simulink model "Noa_Nofusion"  (R2020b)
settings: Solver=FixedStepDiscrete  StartTime=0.0  StopTime=Inf  FixedStep=0.01  RelTol=1e-3
PostLoadFcn:
  | if any(exist('dsrtsu_mdlpostloadfcn', 'file') ~= 0), dsrtsu_mdlpostloadfcn('Execute', bdroot); end
InitFcn:
  | , if any(exist('rtifpga_mdlclblib', 'file') ~= 0), rtifpga_mdlclblib('Init', bdroot); end,
  | , if any(exist('dsmpb_private', 'file') ~= 0), dsmpb_private('dsmpb_mdlclblib', 'Init', bdroot); end,
undefined symbols (not defined in the file or in its folder): ACC_TimeGap_DecSetSwt, ACC_TimeGap_IncSetSwt, AccelPedalPosn, AccelPedalPosnVldty, AccelPedlPosnDiagc, AccPedalOverride, ACU_ShiftInProgress, ADAS_Posn_CurLane, AESSwtReq, ALC_SwtReq, BrkPedalSts, CC_ACC_CANCEL_OFFSwt, CC_ACC_CRUISE_OFFSwt, CC_ACC_DecSetSpd_SetSwt, CC_ACC_IncSetSpd_ResuSwt, CC_ACCSwtErr, CharSpd_ms, CSA_NODE, CURRENT_GEAR, CurrentGearValid, DiscIntNeverNeededParam, DrvDoorSts, DrvSBR, DrvTrqReqOvld, ECMACCInterface, ECMRespACC, ELKSwtReq, EngLimpHomeSts, EngSpd, EngState, EngState_PHEV, EngTrqMaxActSpd, EngTrqMinAct, EPS_DrvInpTrqVal_HighReslolution, EPS_FailSts, EPS_LKATorqOvrlDlvd, EPS_LKATorqOvrlDlvdVld, EPS_LKATrqOvlDlvdSts, EPS_SteerMod, EPS_TrqSnsrSts, EQ4_APPINFO, EQ4_LA_ELEM, EQ4_LA_HDR, EQ4_LAP_ELEM, EQ4_LAP_HDR, EQ4_LH_ELEM, EQ4_LH_HDR, EQ4_LRE_ELEM, EQ4_LRE_HDR, ESS_PedSwtReq, ESS_VehSwtReq, FFogLmpSts_F_Pbox, FLWheelDriveDirection, FLWheelSpd, FrntWiprSwtSts, FrntWshrSwtSts, FRWheelDriveDirection, FRWheelSpd, HazardLmpSwtSts, HCU_AccelPedalPosn_Diag ... (+151)
libraries: simulink x144, dsmpblib x33, canfdmsglib x10
(part 17 of 20)

== matlab function Noa_Nofusion/TOS2/Subsystem1/ACCOSM/HWA_Task100ms1/VycCalc ==
  data: ObjVyc output single size=15; dxC0 input; aP0 input; bP0 input; aP1 input; bP1 input; ObjValid input boolean size=15; ObjDx input single size=15; ObjVxG input single size=15; ObjVyG input single size=15; ObjYawAngle output
function [ObjVyc,ObjYawAngle] = VycCalc(dxC0,aP0,bP0,aP1,bP1,ObjValid,ObjDx,ObjVxG,ObjVyG)

ObjVyc = single(zeros(15,1));
ObjYawAngle = single(zeros(15,1));

for i=1:15
    if ObjValid(i)
       t_dxv = ObjDx(i);
       t_VxG = ObjVxG(i);
       t_VyG = ObjVyG(i);
       
       if abs(t_VxG)<0.1
          if t_VyG>0.5
              ObjYawAngle(i) = single(1.57);
          end
          if t_VyG<-0.5
              ObjYawAngle(i) = single(-1.57);
          end
       else
           if t_VxG>0
               ObjYawAngle(i) = atan(t_VyG/t_VxG);
           else
               if t_VyG>0
                  ObjYawAngle(i) = single(3.1416) + atan(t_VyG/t_VxG);
               else
                  ObjYawAngle(i) = -single(3.1416) + atan(t_VyG/t_VxG);
               end
           end
       end
       
       t_bParabolaYNLane = single(1);
       if t_dxv<dxC0
          temp1 =  2*aP0*t_dxv + bP0;
          t_bParabolaXNLane = -temp1;
       else
          temp1 =  2*aP1*t_dxv + bP1;
          t_bParabolaXNLane = -temp1;
       end
       t_bParabolaMag = mag(t_bParabolaXNLane,t_bParabolaYNLane);
       t_bParabolaXNLane = t_bParabolaXNLane/t_bParabolaMag;
       t_bParabolaYNLane = t_bParabolaYNLane/t_bParabolaMag;
       temp1 = t_VxG*t_bParabolaXNLane;
       temp2 = t_VyG*t_bParabolaYNLane;
       
       ObjVyc(i) = temp1 + temp2;
    else
       ObjVyc(i) = single(0);
    end
end
end

function out = mag(x,y)
M = max(abs(x),abs(y));
N = min(abs(x),abs(y));
out = M + 0.322*N;
end

== matlab function Noa_Nofusion/TOS2/Subsystem1/ACCOSM/HWA_Task100ms1/dyLaneWidthSteerAdapt ==
  data: kap input; dyLaneAdaptLeft output; dyAdapt input; dyLaneAdaptRight output
function [dyLaneAdaptLeft,dyLaneAdaptRight] = fcn(kap,dyAdapt)

dyLaneAdaptLeft = single(0);
dyLaneAdaptRight = single(0);
if kap>0
    dyLaneAdaptRight = dyAdapt;
end
if kap<0
    dyLaneAdaptLeft = dyAdapt;
end

== matlab function Noa_Nofusion/TOS2/Subsystem1/ACCOSM/HWA_Task100ms1/wCutInVy ==
  data: DycASI output single; ObjValid input boolean size=15; ObjDycCutIn input single size=15; ObjWidth input single size=15; ObjVyc input single size=15; ObjDx input single size=15; ObjDy input single size=15; ObjCnt input uint8 size=15; ObjDycFilt input single size=15; ObjwCutInVyK1 input single size=15; ObjtPrediction4CutIn output single size=15; ObjDycCutInPredict output single size=15; ObjCutIn_b output boolean size=15; ObjwCutInVy output single size=15
function [DycASI,ObjtPrediction4CutIn,ObjDycCutInPredict,ObjCutIn_b,ObjwCutInVy] = ...
    CalcWCutInVy(ObjValid,ObjDycCutIn,ObjWidth,ObjVyc,ObjDx,ObjDy,ObjCnt,...
    ObjDycFilt,ObjwCutInVyK1)
 
ObjwCutInVy = single(zeros(15,1));
ObjtPrediction4CutIn = single(zeros(15,1));
ObjDycCutInPredict = single(zeros(15,1));
DycASI = single(zeros(15,1));
ObjCutIn_b = false(15,1);
 
for i=1:15
    if ObjValid(i)
        dWidth = ObjWidth(i);
        dycASI = ObjDycCutIn(i);
        vyc = ObjVyc(i);
        dx = ObjDx(i);
        dy = ObjDy(i);
        dycFilt = ObjDycFilt(i);
        wCutInVyK1 = ObjwCutInVyK1(i);
  
        temp1 = dycFilt - dycASI;
        if ((dycASI>0)&&(temp1>0.2))||((dycASI<0)&&(temp1<-0.2))
            tauVy = single(1.6);
        else
            tauVy = single(0);
        end
        tauVy = interpolate(single(40),tauVy,single(70),single(0),dx);
        ObjtPrediction4CutIn(i) = tauVy;
        temp1 = vyc*tauVy;
        temp2 = dycASI + temp1;
        
        if (dycASI>0)&&(temp2<0)
            temp2 = single(0);
        else
            if (dycASI<0)&&(temp2>0)
                temp2 = single(0);
            else
                if dycASI==0
                    temp2 = single(0);
                end
            end
        end
        ObjDycCutInPredict(i) = temp2;
        if dycASI>0
            temp1 = temp2 - 0.5*dWidth;
            t_dycASI = max(temp1,single(0));
        else
            temp1 = temp2 + 0.5*dWidth;
            t_dycASI = min(temp1,single(0));
        end
        temp1 = abs(t_dycASI);
        t_wCutInVy = interpolate(single(0),single(1),single(0.7),single(0),temp1);
        if tauVy==0
            t_wCutInVy = single(0);
        end
        
        if dx>0
            fak = abs(dy)/dx; 
        else
            fak = single(0);
        end
        if (ObjCnt(i)<2)||(abs(dy)>=2.4)||(fak>0.25)
           t_wCutInVy = single(0);
        end
       
        temp1 = t_wCutInVy - wCutInVyK1;
        temp1_ub = abs(temp1);
        temp2 = 0.2*temp1_ub;
        if temp1>0
            t_wCutInVy = wCutInVyK1 + temp2;
        else
            t_wCutInVy = wCutInVyK1 - temp2;
        end
        ObjwCutInVy(i) = t_wCutInVy;
        DycASI(i) = t_dycASI;
        if t_wCutInVy>0.7
            ObjCutIn_b(i) = true;
        end
    end
end
end
 
% function out = interpolate(x1,z1,x2,z2,Raw)
% if Raw<=x1
%     out = z1;
% else
%     if Raw>=x2
%         out = z2;
%     else
%         out = z1 + (Raw-x1)*(z2-z1)/(x2-x1);
%     end
% end
% end

== matlab function Noa_Nofusion/TOS2/Subsystem1/ACCOSM/HWA_Task100ms1/wCutOutVy ==
  data: vRef input single size=1; kap input single size=1; tDirIndLeft input single size=1; tDirIndRight input single size=1; ObjValid input boolean size=15; ObjDycCutIn input single size=15; ObjWidth input single size=15; ObjtPrediction4CutOut output single size=15; ObjDycCutOutPredict output single size=15; ObjwCutOutTurnOff output single size=15; ObjVyc input single size=15; ObjDx input single size=15; ObjDy input single size=15; ObjVx input single size=15; ObjVy input single size=15; ObjDyc input single size=15; ObjDrive_b input boolean size=15; ObjCnt input uint8 size=15; ObjDycFilt input single size=15; ObjwCutoutVyK1 input single size=15; ObjwCutoutVy output single size=15
function [ObjtPrediction4CutOut,ObjDycCutOutPredict,ObjwCutOutTurnOff,ObjwCutoutVy] = ...
    CalcWCutOutVy(vRef,kap,tDirIndLeft,tDirIndRight,ObjValid,ObjDycCutIn,ObjWidth,...
    ObjVyc,ObjDx,ObjDy,ObjVx,ObjVy,ObjDyc,ObjDrive_b,ObjCnt,...
    ObjDycFilt,ObjwCutoutVyK1)
 
ObjwCutoutVy = single(zeros(15,1));
ObjtPrediction4CutOut = single(zeros(15,1));
ObjDycCutOutPredict = single(zeros(15,1));
ObjwCutOutTurnOff = single(zeros(15,1));
 
for i=1:15
    if ObjValid(i)
        dWidth = ObjWidth(i);
        dycASI = ObjDycCutIn(i);
        vyc = ObjVyc(i);
        dx = ObjDx(i);
        dy = ObjDy(i);
        vx = ObjVx(i);
        vy = ObjVy(i);
        dyc = ObjDyc(i);
        dycFilt = ObjDycFilt(i);
        wCutoutVyK1 = ObjwCutoutVyK1(i);
        Move_b = ObjDrive_b(i);
        Cnt = ObjCnt(i);
        t_vxTO = vRef + vx;
        t_vxvThreshold = 0.5 - vRef;
        
        temp1 = dycASI - dycFilt;
        if ((dycASI>0)&&(temp1>0.2))||((dycASI<0)&&(temp1<-0.2))
            tauVy = single(1);
        else
            tauVy = single(0);
        end
        tauVy = interpolate(single(40),tauVy,single(70),single(0),dx);
        ObjtPrediction4CutOut(i) = tauVy;
        temp1 = vyc*tauVy;
        temp2 = dycASI + temp1;
        
        if (dycASI>0)&&(temp2<0)
            temp2 = single(0);
        else
            if (dycASI<0)&&(temp2>0)
                temp2 = single(0);
            else
                if dycASI==0
                    temp2 = single(0);
                end
            end
        end
        ObjDycCutOutPredict(i) = temp2;
        if dycASI>0
            temp1 = temp2 + 0.5*dWidth;
            t_dycASI = max(temp1,single(0));
        else
            temp1 = temp2 - 0.5*dWidth;
            t_dycASI = min(temp1,single(0));
        end
        temp1 = abs(t_dycASI);
        t_wCutoutVy = interpolate(single(0),single(0),single(0.7),single(1),temp1);
        if tauVy==0
            t_wCutoutVy = single(0);
        end
        
        temp1 = t_wCutoutVy - wCutoutVyK1;
        temp1_ub = abs(temp1);
        temp2 = 0.2*temp1_ub;
        if temp1>0
            t_wCutoutVy = wCutoutVyK1 + temp2;
        else
            t_wCutoutVy = wCutoutVyK1 - temp2;
        end
        ObjwCutoutVy(i) = t_wCutoutVy;
        if (dx<30)&&(Move_b==true)&&(vRef>0.5)&&(t_vxTO<6)&&(vx>t_vxvThreshold)&&(abs(dyc)>0.5)&&...
        (abs(dy)>0.5)&&(abs(dy)<4)&&(abs(vy)>0.5)&&...
        (((dyc<0)&&(vyc<0)&&(tDirIndRight==0))||((dyc>0)&&(vyc>0)&&(tDirIndLeft==0)))&&...
        (kap>-0.005)&&(kap<0.005)&&...
        (Cnt==7) 
             ObjwCutOutTurnOff(i) = t_wCutoutVy;
        end
    end
end
end

== matlab function Noa_Nofusion/TOS2/Subsystem1/ACCOSM/ObjMatrixTransit/Subsystem/MATLAB Function1 ==
  data: P output uint8; Count input uint8 size=1; ID input uint8 size=20; BrakeLight_b input uint8 size=20; Class input uint8 size=20; LatDis input single size=20; LatVel input single size=20; LongAccel input single size=20; LongDis input single size=20; LongVel input single size=20; Width input single size=20; Age input uint16 size=20; MotionSts input uint8 size=20; ObjValid output boolean size=20; ObjBrakeLightIndic output uint8 size=20; ObjClassification output uint8 size=20; ObjLatPos output single size=20; ObjLatVel output single size=20; ObjLongAccel output single size=20; ObjLongVel output single size=20; ObjWidth output single size=20; ObjCnt output uint8 size=20; ObjMoveSts output uint8 size=20; ObjLongPos output single size=20; ObjIDK1 input uint8 size=20; ObjID output uint8 size=20
function [P,ObjValid,ObjBrakeLightIndic,ObjClassification,...
    ObjLatPos,ObjLatVel,ObjLongAccel,ObjLongVel,...
    ObjWidth,ObjCnt,ObjMoveSts,ObjLongPos,ObjID] =...
    DataT(Count,ID,BrakeLight_b,Class,LatDis,LatVel,LongAccel,LongDis,LongVel,Width,Age,MotionSts,ObjIDK1)

ObjValid = false(20,1);
ObjID = uint8(zeros(20,1));
ObjBrakeLightIndic = uint8(zeros(20,1));
ObjClassification = uint8(zeros(20,1));
ObjLatPos = single(zeros(20,1));
ObjLatVel = single(zeros(20,1));
ObjLongAccel = single(zeros(20,1));
ObjLongPos = single(zeros(20,1));
ObjLongVel = single(zeros(20,1));
ObjWidth = single(zeros(20,1));
ObjCnt = uint8(zeros(20,1));
ObjMoveSts = uint8(zeros(20,1));

T = uint8(zeros(20,1));
P = uint8(zeros(20,1));
Index01 = uint8(zeros(20,1));
Index02 = uint8(zeros(20,1));
M = uint8(0);
N = uint8(0);
w = uint8(0);

for i=uint8(1):Count
    for j=uint8(1):uint8(20)
        if ID(i)==ObjIDK1(j)
            T(j) = i;
            P(i) = j;
        end
    end
end

for j=uint8(1):uint8(20)
    if T(j)==uint8(0)
        if ObjIDK1(j)==uint8(0)
            N = N + uint8(1);
            Index01(N) = j;
        else
            M = M + uint8(1);
            Index02(M) = j;
        end
        ObjValid(j) = false;
    else
        ObjValid(j) = true;
    end
end

for i=uint8(1):Count
    if P(i)==uint8(0)
        w = w + uint8(1);
        if w<=N
            P(i) = Index01(w);
        else
            P(i) = Index02(w - N);
        end
        ObjValid(Index01(w)) = true;
    end
    ObjID(P(i)) = ID(i);
    if BrakeLight_b(i)==uint8(1)
        ObjBrakeLightIndic(P(i)) = uint8(2);
    end
    if Class(i)==uint8(1)||Class(i)==uint8(2)||...
            Class(i)==uint8(3)||Class(i)==uint8(6)
        ObjClassification(P(i)) = uint8(1);
    end
    ObjLatPos(P(i)) = -LatDis(i) - single(0.1);
    ObjLatVel(P(i)) = -LatVel(i);
    ObjLongAccel(P(i)) = LongAccel(i);
    ObjLongPos(P(i)) = LongDis(i);
    ObjLongVel(P(i)) = LongVel(i);
    ObjWidth(P(i)) = Width(i);
    if Age(i)<=255
        ObjCnt(P(i)) = uint8(Age(i)/2) - uint8(1);
    else
        ObjCnt(P(i)) = uint8(127);
    end
    if MotionSts(i)==uint8(1)||MotionSts(i)==uint8(3)
        ObjMoveSts(P(i)) = uint8(1);
    elseif MotionSts(i)==uint8(2)||MotionSts(i)==uint8(5)
        if LongVel(i)>-2.5
            ObjMoveSts(P(i)) = uint8(2);
        else
            ObjMoveSts(P(i)) = uint8(4);
        end
    elseif MotionSts(i)==uint8(4)
        ObjMoveSts(P(i)) = uint8(3);
    end
end
end

== matlab function Noa_Nofusion/Chassis1/CheckSum8Bclc4 ==
  data: Data input; MsgByte output; DataID input
function MsgByte  = CheckSum8B(Data,DataID)
CRC_8_H1D_Tbl =[ 0x00, 0x1d, 0x3a, 0x27, 0x74, 0x69, 0x4e, 0x53, 0xe8, 0xf5, 0xd2, 0xcf, 0x9c, 0x81, 0xa6, 0xbb,...
    0xcd, 0xd0, 0xf7, 0xea, 0xb9, 0xa4, 0x83, 0x9e, 0x25, 0x38, 0x1f, 0x02, 0x51, 0x4c, 0x6b, 0x76, 0x87, 0x9a, 0xbd, 0xa0, 0xf3, 0xee, 0xc9, 0xd4,...
    0x6f, 0x72, 0x55, 0x48, 0x1b, 0x06, 0x21, 0x3c, 0x4a, 0x57, 0x70, 0x6d, 0x3e, 0x23, 0x04, 0x19, 0xa2, 0xbf, 0x98, 0x85, 0xd6, 0xcb, 0xec, 0xf1,...
    0x13, 0x0e, 0x29, 0x34, 0x67, 0x7a, 0x5d, 0x40, 0xfb, 0xe6, 0xc1, 0xdc, 0x8f, 0x92, 0xb5, 0xa8, 0xde, 0xc3, 0xe4, 0xf9, 0xaa, 0xb7, 0x90, 0x8d,...
    0x36, 0x2b, 0x0c, 0x11, 0x42, 0x5f, 0x78, 0x65, 0x94, 0x89, 0xae, 0xb3, 0xe0, 0xfd, 0xda, 0xc7, 0x7c, 0x61, 0x46, 0x5b, 0x08, 0x15, 0x32, 0x2f,...
    0x59, 0x44, 0x63, 0x7e, 0x2d, 0x30, 0x17, 0x0a, 0xb1, 0xac, 0x8b, 0x96, 0xc5, 0xd8, 0xff, 0xe2, 0x26, 0x3b, 0x1c, 0x01, 0x52, 0x4f, 0x68, 0x75,...
    0xce, 0xd3, 0xf4, 0xe9, 0xba, 0xa7, 0x80, 0x9d, 0xeb, 0xf6, 0xd1, 0xcc, 0x9f, 0x82, 0xa5, 0xb8, 0x03, 0x1e, 0x39, 0x24, 0x77, 0x6a, 0x4d, 0x50,...
    0xa1, 0xbc, 0x9b, 0x86, 0xd5, 0xc8, 0xef, 0xf2, 0x49, 0x54, 0x73, 0x6e, 0x3d, 0x20, 0x07, 0x1a, 0x6c, 0x71, 0x56, 0x4b, 0x18, 0x05, 0x22, 0x3f,...
    0x84, 0x99, 0xbe, 0xa3, 0xf0, 0xed, 0xca, 0xd7, 0x35, 0x28, 0x0f, 0x12, 0x41, 0x5c, 0x7b, 0x66, 0xdd, 0xc0, 0xe7, 0xfa, 0xa9, 0xb4, 0x93, 0x8e,...
    0xf8, 0xe5, 0xc2, 0xdf, 0x8c, 0x91, 0xb6, 0xab, 0x10, 0x0d, 0x2a, 0x37, 0x64, 0x79, 0x5e, 0x43, 0xb2, 0xaf, 0x88, 0x95, 0xc6, 0xdb, 0xfc, 0xe1,...
    0x5a, 0x47, 0x60, 0x7d, 0x2e, 0x33, 0x14, 0x09, 0x7f, 0x62, 0x45, 0x58, 0x0b, 0x16, 0x31, 0x2c, 0x97, 0x8a, 0xad, 0xb0, 0xe3, 0xfe, 0xd9, 0xc4];

Segment=uint8(zeros(1,8));

for SegIndex =1:8
    CRC_temp=uint8(0);
    for index = 1:8
        Segment(index)=Data((SegIndex-1)*8+index);
    end
    for index = 1:2
        CRC_temp = bitxor(DataID(SegIndex,index),CRC_temp);
        index1=uint16(CRC_temp)+1;
        CRC_temp = CRC_8_H1D_Tbl(index1);
    end
    for index = 2:8
        CRC_temp = bitxor(Segment(index),CRC_temp);
        index2=uint16(CRC_temp)+1;
        CRC_temp = CRC_8_H1D_Tbl(index2);
    end
    Data(8*SegIndex-7)=CRC_temp;
end
MsgByte=Data;
end

== stateflow chart Noa_Nofusion/TOS2/Subsystem1/ACCOSM/ObjMatrixTransit/Subsystem/Obj ==
  (default) -> (junction 5)
  (junction 5) -> (junction 36) : {i=1;}
  (junction 36) -> (junction 38) [order 1] : [i<21]
  (junction 40) -> (junction 36) : {i=i+1;}
  (junction 36) -> (junction 42) [order 2]
  (junction 38) -> (junction 40) : {id(i) = IFV410_Obj(i).OBJ_ID;
      | confidence(i) = IFV410_Obj(i).OBJ_Existence_Probability;
      | classification(i) = IFV410_Obj(i).OBJ_Object_Class;
      | width(i) = IFV410_Obj(i).OBJ_Width;
      | LongDis(i) = IFV410_Obj(i).OBJ_Long_Distance;
      | LatDis(i) = IFV410_Obj(i).OBJ_Lat_Distance;
      | AbsLongAcc(i) = IFV410_Obj(i).OBJ_Abs_Long_Acc;
      | AbsLongVel(i) = IFV410_Obj(i).OBJ_Abs_Long_Velocity;
      | AbsLatVel(i) = IFV410_Obj(i).OBJ_Abs_Lat_Velocity;
      | BrakeLight(i) = IFV410_Obj(i).OBJ_Brake_Light;
      | Age(i) = IFV410_Obj(i).OBJ_Object_Age;
      | motionSts(i) = IFV410_Obj(i).OBJ_Motion_Status;
      | motionCategory(i) = IFV410_Obj(i).OBJ_Motion_Category;
      | motionOrientation(i) = IFV410_Obj(i).OBJ_Motion_Orientation;}
  data: i local uint8; id output uint8 size=20 =uint8(zeros(20,1)); classification output uint8 size=20 =uint8(zeros(20,1)); AbsLongAcc output single size=20 =single(zeros(20,1)); width output single size=20 =single(zeros(20,1)); AbsLongVel output single size=20 =single(zeros(20,1)); LongDis output single size=20 =single(zeros(20,1)); AbsLatVel output single size=20 =single(zeros(20,1)); LatDis output single size=20 =single(zeros(20,1)); BrakeLight output uint8 size=20 =uint8(zeros(20,1)); Age output uint16 size=20 =uint16(zeros(20,1)); confidence output single size=20 =single(zeros(20,1)); IFV410_Obj input Bus: SPI_EQ4_OBJ_ELEM_BUS size=20; motionSts output uint8 size=20 =uint8(zeros(20,1)); motionCategory output uint8 size=20 =uint8(zeros(20,1)); motionOrientation output uint8 size=20 =uint8(zeros(20,1))

== matlab function Noa_Nofusion/TOS/Subsystem2/ACCOSM/HWA_Task100ms1/dyLaneWidthSteerAdapt ==
  data: kap input; dyLaneAdaptLeft output; dyAdapt input; dyLaneAdaptRight output
function [dyLaneAdaptLeft,dyLaneAdaptRight] = fcn(kap,dyAdapt)

dyLaneAdaptLeft = single(0);
dyLaneAdaptRight = single(0);
if kap>0
    dyLaneAdaptRight = dyAdapt;
end
if kap<0
    dyLaneAdaptLeft = dyAdapt;
end

== matlab function Noa_Nofusion/TOS/Subsystem2/ACCOSM/HWA_Task100ms1/wCutInVy ==
  data: DycASI output single; ObjValid input boolean size=15; ObjDycCutIn input single size=15; ObjWidth input single size=15; ObjVyc input single size=15; ObjDx input single size=15; ObjDy input single size=15; ObjCnt input uint8 size=15; ObjDycFilt input single size=15; ObjwCutInVyK1 input single size=15; ObjtPrediction4CutIn output single size=15; ObjDycCutInPredict output single size=15; ObjCutIn_b output boolean size=15; ObjwCutInVy output single size=15
function [DycASI,ObjtPrediction4CutIn,ObjDycCutInPredict,ObjCutIn_b,ObjwCutInVy] = ...
    CalcWCutInVy(ObjValid,ObjDycCutIn,ObjWidth,ObjVyc,ObjDx,ObjDy,ObjCnt,...
    ObjDycFilt,ObjwCutInVyK1)
 
ObjwCutInVy = single(zeros(15,1));
ObjtPrediction4CutIn = single(zeros(15,1));
ObjDycCutInPredict = single(zeros(15,1));
DycASI = single(zeros(15,1));
ObjCutIn_b = false(15,1);
 
for i=1:15
    if ObjValid(i)
        dWidth = ObjWidth(i);
        dycASI = ObjDycCutIn(i);
        vyc = ObjVyc(i);
        dx = ObjDx(i);
        dy = ObjDy(i);
        dycFilt = ObjDycFilt(i);
        wCutInVyK1 = ObjwCutInVyK1(i);
  
        temp1 = dycFilt - dycASI;
        if ((dycASI>0)&&(temp1>0.2))||((dycASI<0)&&(temp1<-0.2))
            tauVy = single(1.6);
        else
            tauVy = single(0);
        end
        tauVy = interpolate(single(40),tauVy,single(70),single(0),dx);
        ObjtPrediction4CutIn(i) = tauVy;
        temp1 = vyc*tauVy;
        temp2 = dycASI + temp1;
        
        if (dycASI>0)&&(temp2<0)
            temp2 = single(0);
        else
            if (dycASI<0)&&(temp2>0)
                temp2 = single(0);
            else
                if dycASI==0
                    temp2 = single(0);
                end
            end
        end
        ObjDycCutInPredict(i) = temp2;
        if dycASI>0
            temp1 = temp2 - 0.5*dWidth;
            t_dycASI = max(temp1,single(0));
        else
            temp1 = temp2 + 0.5*dWidth;
            t_dycASI = min(temp1,single(0));
        end
        temp1 = abs(t_dycASI);
        t_wCutInVy = interpolate(single(0),single(1),single(0.7),single(0),temp1);
        if tauVy==0
            t_wCutInVy = single(0);
        end
        
        if dx>0
            fak = abs(dy)/dx; 
        else
            fak = single(0);
        end
        if (ObjCnt(i)<2)||(abs(dy)>=2.4)||(fak>0.25)
           t_wCutInVy = single(0);
        end
       
        temp1 = t_wCutInVy - wCutInVyK1;
        temp1_ub = abs(temp1);
        temp2 = 0.2*temp1_ub;
        if temp1>0
            t_wCutInVy = wCutInVyK1 + temp2;
        else
            t_wCutInVy = wCutInVyK1 - temp2;
        end
        ObjwCutInVy(i) = t_wCutInVy;
        DycASI(i) = t_dycASI;
        if t_wCutInVy>0.7
            ObjCutIn_b(i) = true;
        end
    end
end
end
 
% function out = interpolate(x1,z1,x2,z2,Raw)
% if Raw<=x1
%     out = z1;
% else
%     if Raw>=x2
%         out = z2;
%     else
%         out = z1 + (Raw-x1)*(z2-z1)/(x2-x1);
%     end
% end
% end

== matlab function Noa_Nofusion/TOS/Subsystem2/ACCOSM/HWA_Task100ms1/wCutOutVy ==
  data: vRef input single size=1; kap input single size=1; tDirIndLeft input single size=1; tDirIndRight input single size=1; ObjValid input boolean size=15; ObjDycCutIn input single size=15; ObjWidth input single size=15; ObjtPrediction4CutOut output single size=15; ObjDycCutOutPredict output single size=15; ObjwCutOutTurnOff output single size=15; ObjVyc input single size=15; ObjDx input single size=15; ObjDy input single size=15; ObjVx input single size=15; ObjVy input single size=15; ObjDyc input single size=15; ObjDrive_b input boolean size=15; ObjCnt input uint8 size=15; ObjDycFilt input single size=15; ObjwCutoutVyK1 input single size=15; ObjwCutoutVy output single size=15
function [ObjtPrediction4CutOut,ObjDycCutOutPredict,ObjwCutOutTurnOff,ObjwCutoutVy] = ...
    CalcWCutOutVy(vRef,kap,tDirIndLeft,tDirIndRight,ObjValid,ObjDycCutIn,ObjWidth,...
    ObjVyc,ObjDx,ObjDy,ObjVx,ObjVy,ObjDyc,ObjDrive_b,ObjCnt,...
    ObjDycFilt,ObjwCutoutVyK1)
 
ObjwCutoutVy = single(zeros(15,1));
ObjtPrediction4CutOut = single(zeros(15,1));
ObjDycCutOutPredict = single(zeros(15,1));
ObjwCutOutTurnOff = single(zeros(15,1));
 
for i=1:15
    if ObjValid(i)
        dWidth = ObjWidth(i);
        dycASI = ObjDycCutIn(i);
        vyc = ObjVyc(i);
        dx = ObjDx(i);
        dy = ObjDy(i);
        vx = ObjVx(i);
        vy = ObjVy(i);
        dyc = ObjDyc(i);
        dycFilt = ObjDycFilt(i);
        wCutoutVyK1 = ObjwCutoutVyK1(i);
        Move_b = ObjDrive_b(i);
        Cnt = ObjCnt(i);
        t_vxTO = vRef + vx;
        t_vxvThreshold = 0.5 - vRef;
        
        temp1 = dycASI - dycFilt;
        if ((dycASI>0)&&(temp1>0.2))||((dycASI<0)&&(temp1<-0.2))
            tauVy = single(1);
        else
            tauVy = single(0);
        end
        tauVy = interpolate(single(40),tauVy,single(70),single(0),dx);
        ObjtPrediction4CutOut(i) = tauVy;
        temp1 = vyc*tauVy;
        temp2 = dycASI + temp1;
        
        if (dycASI>0)&&(temp2<0)
            temp2 = single(0);
        else
            if (dycASI<0)&&(temp2>0)
                temp2 = single(0);
            else
                if dycASI==0
                    temp2 = single(0);
                end
            end
        end
        ObjDycCutOutPredict(i) = temp2;
        if dycASI>0
            temp1 = temp2 + 0.5*dWidth;
            t_dycASI = max(temp1,single(0));
        else
            temp1 = temp2 - 0.5*dWidth;
            t_dycASI = min(temp1,single(0));
        end
        temp1 = abs(t_dycASI);
        t_wCutoutVy = interpolate(single(0),single(0),single(0.7),single(1),temp1);
        if tauVy==0
            t_wCutoutVy = single(0);
        end
        
        temp1 = t_wCutoutVy - wCutoutVyK1;
        temp1_ub = abs(temp1);
        temp2 = 0.2*temp1_ub;
        if temp1>0
            t_wCutoutVy = wCutoutVyK1 + temp2;
        else
            t_wCutoutVy = wCutoutVyK1 - temp2;
        end
        ObjwCutoutVy(i) = t_wCutoutVy;
        if (dx<30)&&(Move_b==true)&&(vRef>0.5)&&(t_vxTO<6)&&(vx>t_vxvThreshold)&&(abs(dyc)>0.5)&&...
        (abs(dy)>0.5)&&(abs(dy)<4)&&(abs(vy)>0.5)&&...
        (((dyc<0)&&(vyc<0)&&(tDirIndRight==0))||((dyc>0)&&(vyc>0)&&(tDirIndLeft==0)))&&...
        (kap>-0.005)&&(kap<0.005)&&...
        (Cnt==7) 
             ObjwCutOutTurnOff(i) = t_wCutoutVy;
        end
    end
end
end

== matlab function Noa_Nofusion/Chassis1/CheckSum8Bclc1 ==
  data: Data input; MsgByte output; DataID input
function MsgByte  = CheckSum8B(Data,DataID)
CRC_8_H1D_Tbl =[ 0x00, 0x1d, 0x3a, 0x27, 0x74, 0x69, 0x4e, 0x53, 0xe8, 0xf5, 0xd2, 0xcf, 0x9c, 0x81, 0xa6, 0xbb,...
    0xcd, 0xd0, 0xf7, 0xea, 0xb9, 0xa4, 0x83, 0x9e, 0x25, 0x38, 0x1f, 0x02, 0x51, 0x4c, 0x6b, 0x76, 0x87, 0x9a, 0xbd, 0xa0, 0xf3, 0xee, 0xc9, 0xd4,...
    0x6f, 0x72, 0x55, 0x48, 0x1b, 0x06, 0x21, 0x3c, 0x4a, 0x57, 0x70, 0x6d, 0x3e, 0x23, 0x04, 0x19, 0xa2, 0xbf, 0x98, 0x85, 0xd6, 0xcb, 0xec, 0xf1,...
    0x13, 0x0e, 0x29, 0x34, 0x67, 0x7a, 0x5d, 0x40, 0xfb, 0xe6, 0xc1, 0xdc, 0x8f, 0x92, 0xb5, 0xa8, 0xde, 0xc3, 0xe4, 0xf9, 0xaa, 0xb7, 0x90, 0x8d,...
    0x36, 0x2b, 0x0c, 0x11, 0x42, 0x5f, 0x78, 0x65, 0x94, 0x89, 0xae, 0xb3, 0xe0, 0xfd, 0xda, 0xc7, 0x7c, 0x61, 0x46, 0x5b, 0x08, 0x15, 0x32, 0x2f,...
    0x59, 0x44, 0x63, 0x7e, 0x2d, 0x30, 0x17, 0x0a, 0xb1, 0xac, 0x8b, 0x96, 0xc5, 0xd8, 0xff, 0xe2, 0x26, 0x3b, 0x1c, 0x01, 0x52, 0x4f, 0x68, 0x75,...
    0xce, 0xd3, 0xf4, 0xe9, 0xba, 0xa7, 0x80, 0x9d, 0xeb, 0xf6, 0xd1, 0xcc, 0x9f, 0x82, 0xa5, 0xb8, 0x03, 0x1e, 0x39, 0x24, 0x77, 0x6a, 0x4d, 0x50,...
    0xa1, 0xbc, 0x9b, 0x86, 0xd5, 0xc8, 0xef, 0xf2, 0x49, 0x54, 0x73, 0x6e, 0x3d, 0x20, 0x07, 0x1a, 0x6c, 0x71, 0x56, 0x4b, 0x18, 0x05, 0x22, 0x3f,...
    0x84, 0x99, 0xbe, 0xa3, 0xf0, 0xed, 0xca, 0xd7, 0x35, 0x28, 0x0f, 0x12, 0x41, 0x5c, 0x7b, 0x66, 0xdd, 0xc0, 0xe7, 0xfa, 0xa9, 0xb4, 0x93, 0x8e,...
    0xf8, 0xe5, 0xc2, 0xdf, 0x8c, 0x91, 0xb6, 0xab, 0x10, 0x0d, 0x2a, 0x37, 0x64, 0x79, 0x5e, 0x43, 0xb2, 0xaf, 0x88, 0x95, 0xc6, 0xdb, 0xfc, 0xe1,...
    0x5a, 0x47, 0x60, 0x7d, 0x2e, 0x33, 0x14, 0x09, 0x7f, 0x62, 0x45, 0x58, 0x0b, 0x16, 0x31, 0x2c, 0x97, 0x8a, 0xad, 0xb0, 0xe3, 0xfe, 0xd9, 0xc4];

CRC_temp=uint8(zeros(1));

for t_index = 1:2
    CRC_temp = bitxor(DataID(t_index),CRC_temp);
    CRC_temp = CRC_8_H1D_Tbl(CRC_temp+1);
end

for t_index = 10:16
    CRC_temp = bitxor(Data(t_index),CRC_temp);
    CRC_temp = CRC_8_H1D_Tbl(CRC_temp+1);
end
Data(9)=CRC_temp;
MsgByte=Data;
end

== matlab function Noa_Nofusion/TOS/Subsystem2/ACCOSM/ObjMatrixTransit/Subsystem/MATLAB Function1 ==
  data: P output uint8; Count input uint8 size=1; ID input uint8 size=20; BrakeLight_b input uint8 size=20; Class input uint8 size=20; LatDis input single size=20; LatVel input single size=20; LongAccel input single size=20; LongDis input single size=20; LongVel input single size=20; Width input single size=20; Age input uint16 size=20; MotionSts input uint8 size=20; ObjValid output boolean size=20; ObjBrakeLightIndic output uint8 size=20; ObjClass output; ObjClassification output uint8 size=20; ObjLatPos output single size=20; ObjLatVel output single size=20; ObjLongAccel output single size=20; ObjLongVel output single size=20; ObjWidth output single size=20; ObjCnt output uint8 size=20; ObjMoveSts output uint8 size=20; ObjLongPos output single size=20; ObjIDK1 input uint8 size=20; ObjID output uint8 size=20
function [P,ObjValid,ObjBrakeLightIndic,ObjClass,ObjClassification,...
    ObjLatPos,ObjLatVel,ObjLongAccel,ObjLongVel,...
    ObjWidth,ObjCnt,ObjMoveSts,ObjLongPos,ObjID] =...
    DataT(Count,ID,BrakeLight_b,Class,LatDis,LatVel,LongAccel,LongDis,LongVel,Width,Age,MotionSts,ObjIDK1)

ObjValid = false(20,1);
ObjID = uint8(zeros(20,1));
ObjBrakeLightIndic = uint8(zeros(20,1));
ObjClassification = uint8(zeros(20,1));
ObjClass  = uint8(zeros(20,1));
ObjLatPos = single(zeros(20,1));
ObjLatVel = single(zeros(20,1));
ObjLongAccel = single(zeros(20,1));
ObjLongPos = single(zeros(20,1));
ObjLongVel = single(zeros(20,1));
ObjWidth = single(zeros(20,1));
ObjCnt = uint8(zeros(20,1));
ObjMoveSts = uint8(zeros(20,1));

T = uint8(zeros(20,1));
P = uint8(zeros(20,1));
Index01 = uint8(zeros(20,1));
Index02 = uint8(zeros(20,1));
M = uint8(0);
N = uint8(0);
w = uint8(0);

for i=uint8(1):Count
    for j=uint8(1):uint8(20)
        if ID(i)==ObjIDK1(j)
            T(j) = i;
            P(i) = j;
        end
    end
end

for j=uint8(1):uint8(20)
    if T(j)==uint8(0)
        if ObjIDK1(j)==uint8(0)
            N = N + uint8(1);
            Index01(N) = j;
        else
            M = M + uint8(1);
            Index02(M) = j;
        end
        ObjValid(j) = false;
    else
        ObjValid(j) = true;
    end
end

for i=uint8(1):Count
    if P(i)==uint8(0)
        w = w + uint8(1);
        if w<=N
            P(i) = Index01(w);
        else
            P(i) = Index02(w - N);
        end
        ObjValid(Index01(w)) = true;
    end
    ObjID(P(i)) = ID(i);
    if BrakeLight_b(i)==uint8(1)
        ObjBrakeLightIndic(P(i)) = uint8(2);
    end
    if Class(i)==uint8(1)||Class(i)==uint8(2)||...
            Class(i)==uint8(3)||Class(i)==uint8(6)
        ObjClassification(P(i)) = uint8(1);
    end
    ObjClass(P(i)) = uint8(Class(i));
    ObjLatPos(P(i)) = -LatDis(i) - single(0.1);
    ObjLatVel(P(i)) = -LatVel(i);
    ObjLongAccel(P(i)) = LongAccel(i);
    ObjLongPos(P(i)) = LongDis(i);
    ObjLongVel(P(i)) = LongVel(i);
    ObjWidth(P(i)) = Width(i);
    if Age(i)<=255
        ObjCnt(P(i)) = uint8(Age(i)/2) - uint8(1);
    else
        ObjCnt(P(i)) = uint8(127);
    end
    if MotionSts(i)==uint8(1)||MotionSts(i)==uint8(3)
        ObjMoveSts(P(i)) = uint8(1);
    elseif MotionSts(i)==uint8(2)||MotionSts(i)==uint8(5)
        if LongVel(i)>-2.5
            ObjMoveSts(P(i)) = uint8(2);
        else
            ObjMoveSts(P(i)) = uint8(4);
        end
    elseif MotionSts(i)==uint8(4)
        ObjMoveSts(P(i)) = uint8(3);
    end
end
end

== stateflow chart Noa_Nofusion/TOS/Subsystem2/ACCOSM/ObjMatrixTransit/Subsystem/Obj ==
  (default) -> (junction 5)
  (junction 5) -> (junction 36) : {i=1;}
  (junction 36) -> (junction 38) [order 1] : [i<21]
  (junction 40) -> (junction 36) : {i=i+1;}
  (junction 36) -> (junction 42) [order 2]
  (junction 38) -> (junction 40) : {id(i) = IFV410_Obj(i).OBJ_ID;
      | confidence(i) = IFV410_Obj(i).OBJ_Existence_Probability;
      | classification(i) = IFV410_Obj(i).OBJ_Object_Class;
      | width(i) = IFV410_Obj(i).OBJ_Width;
      | LongDis(i) = IFV410_Obj(i).OBJ_Long_Distance;
      | LatDis(i) = IFV410_Obj(i).OBJ_Lat_Distance;
      | AbsLongAcc(i) = IFV410_Obj(i).OBJ_Abs_Long_Acc;
      | AbsLongVel(i) = IFV410_Obj(i).OBJ_Abs_Long_Velocity;
      | AbsLatVel(i) = IFV410_Obj(i).OBJ_Abs_Lat_Velocity;
      | BrakeLight(i) = IFV410_Obj(i).OBJ_Brake_Light;
      | Age(i) = IFV410_Obj(i).OBJ_Object_Age;
      | motionSts(i) = IFV410_Obj(i).OBJ_Motion_Status;
      | motionCategory(i) = IFV410_Obj(i).OBJ_Motion_Category;
      | motionOrientation(i) = IFV410_Obj(i).OBJ_Motion_Orientation;}
  data: i local uint8; id output uint8 size=20 =uint8(zeros(20,1)); classification output uint8 size=20 =uint8(zeros(20,1)); AbsLongAcc output single size=20 =single(zeros(20,1)); width output single size=20 =single(zeros(20,1)); AbsLongVel output single size=20 =single(zeros(20,1)); LongDis output single size=20 =single(zeros(20,1)); AbsLatVel output single size=20 =single(zeros(20,1)); LatDis output single size=20 =single(zeros(20,1)); BrakeLight output uint8 size=20 =uint8(zeros(20,1)); Age output uint16 size=20 =uint16(zeros(20,1)); confidence output single size=20 =single(zeros(20,1)); IFV410_Obj input Bus: SPI_EQ4_OBJ_ELEM_BUS size=20; motionSts output uint8 size=20 =uint8(zeros(20,1)); motionCategory output uint8 size=20 =uint8(zeros(20,1)); motionOrientation output uint8 size=20 =uint8(zeros(20,1))

== matlab function Noa_Nofusion/Chassis1/CheckSum8Bclc2 ==
  data: Data input; MsgByte output; DataID input
function MsgByte  = CheckSum8B(Data,DataID)
CRC_8_H1D_Tbl =[ 0x00, 0x1d, 0x3a, 0x27, 0x74, 0x69, 0x4e, 0x53, 0xe8, 0xf5, 0xd2, 0xcf, 0x9c, 0x81, 0xa6, 0xbb,...
    0xcd, 0xd0, 0xf7, 0xea, 0xb9, 0xa4, 0x83, 0x9e, 0x25, 0x38, 0x1f, 0x02, 0x51, 0x4c, 0x6b, 0x76, 0x87, 0x9a, 0xbd, 0xa0, 0xf3, 0xee, 0xc9, 0xd4,...
    0x6f, 0x72, 0x55, 0x48, 0x1b, 0x06, 0x21, 0x3c, 0x4a, 0x57, 0x70, 0x6d, 0x3e, 0x23, 0x04, 0x19, 0xa2, 0xbf, 0x98, 0x85, 0xd6, 0xcb, 0xec, 0xf1,...
    0x13, 0x0e, 0x29, 0x34, 0x67, 0x7a, 0x5d, 0x40, 0xfb, 0xe6, 0xc1, 0xdc, 0x8f, 0x92, 0xb5, 0xa8, 0xde, 0xc3, 0xe4, 0xf9, 0xaa, 0xb7, 0x90, 0x8d,...
    0x36, 0x2b, 0x0c, 0x11, 0x42, 0x5f, 0x78, 0x65, 0x94, 0x89, 0xae, 0xb3, 0xe0, 0xfd, 0xda, 0xc7, 0x7c, 0x61, 0x46, 0x5b, 0x08, 0x15, 0x32, 0x2f,...
    0x59, 0x44, 0x63, 0x7e, 0x2d, 0x30, 0x17, 0x0a, 0xb1, 0xac, 0x8b, 0x96, 0xc5, 0xd8, 0xff, 0xe2, 0x26, 0x3b, 0x1c, 0x01, 0x52, 0x4f, 0x68, 0x75,...
    0xce, 0xd3, 0xf4, 0xe9, 0xba, 0xa7, 0x80, 0x9d, 0xeb, 0xf6, 0xd1, 0xcc, 0x9f, 0x82, 0xa5, 0xb8, 0x03, 0x1e, 0x39, 0x24, 0x77, 0x6a, 0x4d, 0x50,...
    0xa1, 0xbc, 0x9b, 0x86, 0xd5, 0xc8, 0xef, 0xf2, 0x49, 0x54, 0x73, 0x6e, 0x3d, 0x20, 0x07, 0x1a, 0x6c, 0x71, 0x56, 0x4b, 0x18, 0x05, 0x22, 0x3f,...
    0x84, 0x99, 0xbe, 0xa3, 0xf0, 0xed, 0xca, 0xd7, 0x35, 0x28, 0x0f, 0x12, 0x41, 0x5c, 0x7b, 0x66, 0xdd, 0xc0, 0xe7, 0xfa, 0xa9, 0xb4, 0x93, 0x8e,...
    0xf8, 0xe5, 0xc2, 0xdf, 0x8c, 0x91, 0xb6, 0xab, 0x10, 0x0d, 0x2a, 0x37, 0x64, 0x79, 0x5e, 0x43, 0xb2, 0xaf, 0x88, 0x95, 0xc6, 0xdb, 0xfc, 0xe1,...
    0x5a, 0x47, 0x60, 0x7d, 0x2e, 0x33, 0x14, 0x09, 0x7f, 0x62, 0x45, 0x58, 0x0b, 0x16, 0x31, 0x2c, 0x97, 0x8a, 0xad, 0xb0, 0xe3, 0xfe, 0xd9, 0xc4];

Segment=uint8(zeros(1,8));

for SegIndex =1:8
    CRC_temp=uint8(0);
    for index = 1:8
        Segment(index)=Data((SegIndex-1)*8+index);
    end
    for index = 1:2
        CRC_temp = bitxor(DataID(SegIndex,index),CRC_temp);
        index1=uint16(CRC_temp)+1;
        CRC_temp = CRC_8_H1D_Tbl(index1);
    end
    for index = 2:8
        CRC_temp = bitxor(Segment(index),CRC_temp);
        index2=uint16(CRC_temp)+1;
        CRC_temp = CRC_8_H1D_Tbl(index2);
    end
    Data(8*SegIndex-7)=CRC_temp;
end
MsgByte=Data;
end

== matlab function Noa_Nofusion/TOS/Subsystem2/Subsystem/MATLAB Function1 ==
  data: ObjID input uint8; Dx output single; ObjDy input single; ObjDx input single; ObjVx input single; Dy output single; Vx output single; ID output uint8; Width output single; Class output uint8; FusType output uint8
function [Dx,Dy,Vx,ID,Width,Class,FusType] = fcn(ObjID,ObjDy,ObjDx,ObjVx)

t_dx = single(-255*ones(6,1));
FirObjID = uint8(0);
FirObjDx = single(-255);
SecObjID = uint8(0);
SecObjDx = single(-255);
Dx = single(zeros(2,1));
Dy = single(zeros(2,1));
Vx = single(zeros(2,1));
ID = uint8(zeros(2,1));
Width = single(zeros(2,1));
Class = uint8(zeros(2,1));
FusType = uint8(zeros(2,1));

for i = 1:6
    if ObjID(i)>0
        t_y = ObjDy(i);
        if t_y >1.5 && t_y <5
            t_dx(i) = ObjDx(i);
        end
    end
end
for j = 1:6
    if t_dx(j)> -100
        if t_dx(j) > FirObjDx
            SecObjID =  FirObjID;
            SecObjDx = FirObjDx;
            FirObjID =  uint8(j);
            FirObjDx =  t_dx(j);
        elseif (t_dx(j)>SecObjDx)
            SecObjID = uint8(j);
            SecObjDx = t_dx(j);
        end
    end
end

if FirObjID >0
    Dx(1) = ObjDx(FirObjID);
    Dy(1) = ObjDy(FirObjID);
    Vx(1) = ObjVx(FirObjID);
    ID(1) = uint8(3);
    Width(1) = single(2.1);
    Class(1) = uint8(2);
    FusType(1) = uint8(3);
end
if SecObjID >0
    Dx(2) = ObjDx(SecObjID);
    Dy(2) = ObjDy(SecObjID);
    Vx(2) = ObjVx(SecObjID);
    ID(2) = uint8(4);
    Width(2) = single(2.1);
    Class(2) = uint8(2);
    FusType(2) = uint8(3);
end
        
        










%     k = 6;
%      while (k >j)
%         if t_dx(k)> t_dx(k-1)
%             t_h = t_dx(k);
%             t_dx(k)= t_dx(k-1);
%             t_dx(k-1) = t_h;
%         end
%         k = k-uint8(1);
%      end
% end
% for h = 1:2
%     if

== matlab function Noa_Nofusion/TOS/Subsystem2/Subsystem/MATLAB Function2 ==
  data: ObjID input uint8; Dx output single; ObjDy input single; ObjDx input single; ObjVx input single; Dy output single; Vx output single; ID output uint8; Width output single; Class output uint8; FusType output uint8
function [Dx,Dy,Vx,ID,Width,Class,FusType] = fcn(ObjID,ObjDy,ObjDx,ObjVx)

t_dx = single(-255*ones(6,1));
FirObjID = uint8(0);
FirObjDx = single(-255);
SecObjID = uint8(0);
SecObjDx = single(-255);
Dx = single(zeros(2,1));
Dy = single(zeros(2,1));
Vx = single(zeros(2,1));
ID = uint8(zeros(2,1));
Width = single(zeros(2,1));
Class = uint8(zeros(2,1));
FusType = uint8(zeros(2,1));

for i = 1:6
    if ObjID(i)>0
        t_y = ObjDy(i);
        if t_y <-1.5 && t_y >-5
            t_dx(i) = ObjDx(i);
        end
    end
end
for j = 1:6
    if t_dx(j)> -100
        if t_dx(j) > FirObjDx
            SecObjID =  FirObjID;
            SecObjDx = FirObjDx;
            FirObjID =  uint8(j);
            FirObjDx =  t_dx(j);
        elseif (t_dx(j)>SecObjDx)
            SecObjID = uint8(j);
            SecObjDx = t_dx(j);
        end
    end
end

if FirObjID >0
    Dx(1) = ObjDx(FirObjID);
    Dy(1) = ObjDy(FirObjID);
    Vx(1) = ObjVx(FirObjID);
    ID(1) = uint8(7);
    Width(1) = single(2.1);
    Class(1) = uint8(2);
    FusType(1) = uint8(3);
end
if SecObjID >0
    Dx(2) = ObjDx(SecObjID);
    Dy(2) = ObjDy(SecObjID);
    Vx(2) = ObjVx(SecObjID);
    ID(2) = uint8(8);
    Width(2) = single(2.1);
    Class(2) = uint8(2);
    FusType(2) = uint8(3);
end
        
        










%     k = 6;
%      while (k >j)
%         if t_dx(k)> t_dx(k-1)
%             t_h = t_dx(k);
%             t_dx(k)= t_dx(k-1);
%             t_dx(k-1) = t_h;
%         end
%         k = k-uint8(1);
%      end
% end
% for h = 1:2
%     if

== matlab function Noa_Nofusion/TOS/Subsystem2/Subsystem/MATLAB Function3 ==
  data: ObjID input uint8; Dx output single; ObjDy input single; ObjDx input single; ObjVx input single; ObjClass input; Dy output single; Vx output single; ID output uint8; Width output single; Class output uint8; FusType output uint8; L_Valid input; C0 input; C1 input; C2 input; C3 input; vxv input
function [Dx,Dy,Vx,ID,Width,Class,FusType] = fcn(ObjID,ObjDy,ObjDx,ObjVx,ObjClass,L_Valid,C0,C1,C2,C3,vxv)


Dx = single(zeros(5,1));
Dy = single(zeros(5,1));
Vx = single(zeros(5,1));
ID = uint8(zeros(5,1));
Width = single(zeros(5,1));
Class = uint8(zeros(5,1));
FusType = uint8(zeros(5,1));

ObjLine = uint8(zeros(20,1));
FirObjID_L = uint8(0);
FirObjDx_L = single(255);
SecObjID_L = uint8(0);
SecObjDx_L = single(255);
FirObjID_R = uint8(0);
FirObjDx_R = single(255);
SecObjID_R = uint8(0);
SecObjDx_R = single(255);
FirObjID_E = uint8(0);
FirObjDx_E = single(255);
 
 
 
 
 

for i = 1:20
   if ObjID(i)>0 && L_Valid >0.5
       t_x = ObjDx(i);
       t_y = ObjDy(i);
       t_yC = C0 + C1*t_x + C2*t_x^2 + C3*t_x^3;
       kC = C1+ 2*C2*t_x + 3*C3*t_x^2;
       t_k = sqrt(kC^2+1);
       detaY = (t_y - t_yC)/t_k;
       if detaY > 2 && detaY < 5
           ObjLine(i)=uint8(1);
       elseif detaY < -2 && detaY > -5
           ObjLine(i)=uint8(2);
       elseif detaY < 2 && detaY > -2
           ObjLine(i)=uint8(3);
       end
   end
end

for j = 1:20
    t_x = ObjDx(i);
    if  ObjLine(j)==1 && t_x > -1
        if t_x < FirObjDx_L
            SecObjID_L =  FirObjID_L;
            SecObjDx_L = FirObjDx_L;
            FirObjID_L =  uint8(j);
            FirObjDx_L =  t_x;
        elseif (t_x < SecObjDx_L)
            SecObjID_L = uint8(j);
            SecObjDx_L = t_x;
        end
    elseif ObjLine(j)==2
        if t_x < FirObjDx_R
            SecObjID_R =  FirObjID_R;
            SecObjDx_R = FirObjDx_R;
            FirObjID_R =  uint8(j);
            FirObjDx_R =  t_x;
        elseif (t_x<SecObjDx_R)
            SecObjID_R = uint8(j);
            SecObjDx_R = t_x;
        end
    elseif ObjLine(j)==3
         if t_x < FirObjDx_E
             FirObjID_E =  uint8(j);
             FirObjDx_E =  t_x;
         end
    end
end

if FirObjID_L >0
    Dx(1) = ObjDx(FirObjID_L);
    Dy(1) = ObjDy(FirObjID_L);
    Vx(1) = ObjVx(FirObjID_L)-vxv;
    ID(1) = uint8(1);
    Width(1) = single(2.1);
    Class(1) = ObjClass(FirObjID_L)+uint8(1);
    FusType(1) = uint8(3);
end
if SecObjID_L >0
    Dx(2) = ObjDx(SecObjID_L);
    Dy(2) = ObjDy(SecObjID_L);
    Vx(2) = ObjVx(SecObjID_L)-vxv;
    ID(2) = uint8(2);
    Width(2) = single(2.1);
    Class(2) = ObjClass(SecObjID_L)+uint8(1);
    FusType(2) = uint8(3);
end 
if FirObjID_R >0
    Dx(3) = ObjDx(FirObjID_R);
    Dy(3) = ObjDy(FirObjID_R);
    Vx(3) = ObjVx(FirObjID_R)-vxv;
    ID(3) = uint8(5);
    Width(3) = single(2.1);
    Class(3) =  ObjClass(FirObjID_R)+uint8(1);
    FusType(3) = uint8(3);
end
if SecObjID_R >0
    Dx(4) = ObjDx(SecObjID_R);
    Dy(4) = ObjDy(SecObjID_R);
    Vx(4) = ObjVx(SecObjID_R)-vxv;
    ID(4) = uint8(6);
    Width(4) = single(2.1);
    Class(4) =  ObjClass(SecObjID_R)+uint8(1);
    FusType(4) = uint8(3);
end 
if FirObjID_E >0
    Dx(5) = ObjDx(FirObjID_E);
    Dy(5) = ObjDy(FirObjID_E);
    Vx(5) = ObjVx(FirObjID_E)-vxv;
    ID(5) = uint8(9);
    Width(5) = single(2.1);
    Class(5) = ObjClass(FirObjID_E)+uint8(1);
    FusType(5) = uint8(3);
end
        
           
       




%     k = 6;
%      while (k >j)
%         if t_dx(k)> t_dx(k-1)
%             t_h = t_dx(k);
%             t_dx(k)= t_dx(k-1);
%             t_dx(k-1) = t_h;
%         end
%         k = k-uint8(1);
%      end
% end
% for h = 1:2
%     if

== matlab function Noa_Nofusion/TOS/Subsystem2/DOP/HWA_Task100ms1/Plaus ==
  data: dxMaxFollow input single size=1; ObjValid input boolean size=15; ObjDx input single size=15; ObjVx input single size=15; ObjPlaus output single size=15; ObjOnLeft input single size=15; ObjPlausLeft output single size=15; ObjPlausRight output single size=15; ObjOnRight input single size=15; ObjDycHist input single size=15; ObjqDycHist input single size=15; ObjLpb input single size=15; ObjLpbLeft input single size=15; ObjLpbRight input single size=15; ObjPlausK1 input single size=15; ObjPlausLeftK1 input single size=15; ObjPlausRightK1 input single size=15
function [ObjPlaus,ObjPlausLeft,ObjPlausRight] = ...
    PlausCalc(dxMaxFollow,ObjValid,ObjDx,ObjVx,ObjOnLeft,ObjOnRight,ObjDycHist,ObjqDycHist,...
    ObjLpb,ObjLpbLeft,ObjLpbRight,ObjPlausK1,ObjPlausLeftK1,ObjPlausRightK1)

[ObjPlaus,ObjPlausLeft,ObjPlausRight] = ...
    PlausCalc(dxMaxFollow,ObjValid,ObjDx,ObjVx,ObjOnLeft,ObjOnRight,ObjDycHist,ObjqDycHist,...
    ObjLpb,ObjLpbLeft,ObjLpbRight,ObjPlausK1,ObjPlausLeftK1,ObjPlausRightK1);
end

== matlab function Noa_Nofusion/TOS/Subsystem2/DOP/HWA_Task100ms1/Spw ==
  data: AlpSumSlideCurveness input single size=1; kapCourseErr input single size=1; ObjSpw output single size=15; ObjValid input boolean size=15; DycASI input single size=15; ObjDx input single size=15; ObjSpwLeft output single size=15; ObjSpwRight output single size=15; ObjOnLeft output; ObjOnRight output; ObjDyc input; ObjDycHist input; ObjqDycHist input; ObjDycASI output; ObjDyKapErr output
function [ObjSpw,ObjSpwLeft,ObjSpwRight,ObjOnLeft,ObjOnRight,ObjDycASI,ObjDyKapErr] = ...
    CalcSpw(AlpSumSlideCurveness,kapCourseErr,ObjValid,DycASI,ObjDx,ObjDyc,ObjDycHist,ObjqDycHist)
 
ObjSpw = single(zeros(15,1));
ObjSpwLeft = single(zeros(15,1));
ObjSpwRight = single(zeros(15,1));
ObjOnLeft = single(zeros(15,1));
ObjOnRight = single(zeros(15,1));
ObjDycASI = single(zeros(15,1));
ObjDyKapErr = single(zeros(15,1));
 
for i=1:15
    if ObjValid(i)
        t_dycASI = DycASI(i);
        t_kapErrMin = single(0.0002);
        t_kapErrCurvenessMax = single(0.0018);
        
        temp1 = min(AlpSumSlideCurveness,single(1));
        t_kapErrCurveness = t_kapErrCurvenessMax*temp1;
        t_kapErr = max(t_kapErrMin,max(kapCourseErr,t_kapErrCurveness));
        temp1 = min(ObjDx(i),single(80));
        t_DyKapErr = t_kapErr*temp1*temp1/2;
        ObjDyKapErr(i) = t_DyKapErr;
        
        %         t_dyHalfLane = 1.5;
        %         t_dy3halfLane = 5.25;
        
        if abs(t_dycASI)>=4.5
            t_spw = single(0);
            t_spwNeighbour = single(0);
        elseif abs(t_dycASI)>=3
            t_spw = single(0);
            t_dycToLane = abs(t_dycASI) - single(3);
            t_spwNeighbour = CalcSPW(t_dycToLane,single(3),t_DyKapErr);
        elseif abs(t_dycASI)>=1.5
            t_spw = single(0);
            t_spwNeighbour = CalcSPW(single(0),single(3),t_DyKapErr);
        else
            t_spwNeighbour = single(0);
            t_spw = CalcSPW(single(0),single(3),t_DyKapErr);
        end
        if t_dycASI>=0
            t_spwRight = single(0);
            t_spwLeft = t_spwNeighbour;
        else
            t_spwLeft = single(0);
            t_spwRight = t_spwNeighbour;
        end
        ObjSpw(i) = t_spw;
        ObjSpwLeft(i) = t_spwLeft;
        ObjSpwRight(i) = t_spwRight;
        % -------------------------------------------------------------------------
        
        temp1 = 0.5*ObjqDycHist(i);
        t_dycASI = ObjDyc(i)*(1-temp1) + ObjDycHist(i)*temp1;
        temp2 = single(1.5) + t_DyKapErr;
        temp3 = single(3) + t_DyKapErr;
        ObjDycASI(i) = t_dycASI;
        
        if t_dycASI>=0
            temp1 = max(single(1.5),min(temp3,t_dycASI)) - single(1.5);
            ObjOnLeft(i) = min(single(1),temp1/temp2);
        else
            temp1 = max(min(single(-1.5),t_dycASI),-temp3);
            temp1 = -temp1 - single(1.5);
            ObjOnRight(i) = min(single(1),temp1/temp2);
        end
    end
end
end
 
function t_spw = CalcSPW(absDyc,dyLaneWidth,dyKapErr)
temp3 = dyLaneWidth/2;
temp1 = temp3 - dyKapErr;
temp2 = temp3 + dyKapErr;
temp2 = min(temp2,dyLaneWidth);
 
if absDyc<=temp1
    t_spw = single(1);
elseif absDyc>=temp2
    t_spw = single(0);
else
    temp3 = temp2 - absDyc;
    temp4 = 2*dyKapErr;
    t_spw = temp3/temp4;
end
end

== matlab function Noa_Nofusion/Chassis1/CheckSum8Bclc3 ==
  data: Data input; MsgByte output; DataID input
function MsgByte  = CheckSum8B(Data,DataID)
CRC_8_H1D_Tbl =[ 0x00, 0x1d, 0x3a, 0x27, 0x74, 0x69, 0x4e, 0x53, 0xe8, 0xf5, 0xd2, 0xcf, 0x9c, 0x81, 0xa6, 0xbb,...
    0xcd, 0xd0, 0xf7, 0xea, 0xb9, 0xa4, 0x83, 0x9e, 0x25, 0x38, 0x1f, 0x02, 0x51, 0x4c, 0x6b, 0x76, 0x87, 0x9a, 0xbd, 0xa0, 0xf3, 0xee, 0xc9, 0xd4,...
    0x6f, 0x72, 0x55, 0x48, 0x1b, 0x06, 0x21, 0x3c, 0x4a, 0x57, 0x70, 0x6d, 0x3e, 0x23, 0x04, 0x19, 0xa2, 0xbf, 0x98, 0x85, 0xd6, 0xcb, 0xec, 0xf1,...
    0x13, 0x0e, 0x29, 0x34, 0x67, 0x7a, 0x5d, 0x40, 0xfb, 0xe6, 0xc1, 0xdc, 0x8f, 0x92, 0xb5, 0xa8, 0xde, 0xc3, 0xe4, 0xf9, 0xaa, 0xb7, 0x90, 0x8d,...
    0x36, 0x2b, 0x0c, 0x11, 0x42, 0x5f, 0x78, 0x65, 0x94, 0x89, 0xae, 0xb3, 0xe0, 0xfd, 0xda, 0xc7, 0x7c, 0x61, 0x46, 0x5b, 0x08, 0x15, 0x32, 0x2f,...
    0x59, 0x44, 0x63, 0x7e, 0x2d, 0x30, 0x17, 0x0a, 0xb1, 0xac, 0x8b, 0x96, 0xc5, 0xd8, 0xff, 0xe2, 0x26, 0x3b, 0x1c, 0x01, 0x52, 0x4f, 0x68, 0x75,...
    0xce, 0xd3, 0xf4, 0xe9, 0xba, 0xa7, 0x80, 0x9d, 0xeb, 0xf6, 0xd1, 0xcc, 0x9f, 0x82, 0xa5, 0xb8, 0x03, 0x1e, 0x39, 0x24, 0x77, 0x6a, 0x4d, 0x50,...
    0xa1, 0xbc, 0x9b, 0x86, 0xd5, 0xc8, 0xef, 0xf2, 0x49, 0x54, 0x73, 0x6e, 0x3d, 0x20, 0x07, 0x1a, 0x6c, 0x71, 0x56, 0x4b, 0x18, 0x05, 0x22, 0x3f,...
    0x84, 0x99, 0xbe, 0xa3, 0xf0, 0xed, 0xca, 0xd7, 0x35, 0x28, 0x0f, 0x12, 0x41, 0x5c, 0x7b, 0x66, 0xdd, 0xc0, 0xe7, 0xfa, 0xa9, 0xb4, 0x93, 0x8e,...
    0xf8, 0xe5, 0xc2, 0xdf, 0x8c, 0x91, 0xb6, 0xab, 0x10, 0x0d, 0x2a, 0x37, 0x64, 0x79, 0x5e, 0x43, 0xb2, 0xaf, 0x88, 0x95, 0xc6, 0xdb, 0xfc, 0xe1,...
    0x5a, 0x47, 0x60, 0x7d, 0x2e, 0x33, 0x14, 0x09, 0x7f, 0x62, 0x45, 0x58, 0x0b, 0x16, 0x31, 0x2c, 0x97, 0x8a, 0xad, 0xb0, 0xe3, 0xfe, 0xd9, 0xc4];
Segment=uint8(zeros(1,8));

for SegIndex =1:8
    CRC_temp=uint8(0);
    for index = 1:8
        Segment(index)=Data((SegIndex-1)*8+index);
    end
    for index = 1:2
        CRC_temp = bitxor(DataID(SegIndex,index),CRC_temp);
        index1=uint16(CRC_temp)+1;
        CRC_temp = CRC_8_H1D_Tbl(index1);
    end
    for index = 2:8
        CRC_temp = bitxor(Segment(index),CRC_temp);
        index2=uint16(CRC_temp)+1;
        CRC_temp = CRC_8_H1D_Tbl(index2);
    end
    Data(8*SegIndex-7)=CRC_temp;
end
MsgByte=Data;
end

== matlab function Noa_Nofusion/TOS/Subsystem2/DOP/HWA_Task100ms1/Std ==
  data: u input; y output
function y = fcn(u)

y = std(u);

== matlab function Noa_Nofusion/TOS/Subsystem2/DOP/HWA_Task100ms1/TargetBrake ==
  data: ID input uint8; VxG input; VyG input; TargetBrake_b output boolean; TargetVxG output; BrakeLightIndic input uint8 size=15; TargetVyG output
function [TargetBrake_b,TargetVxG,TargetVyG] = fcn(ID,VxG,VyG,BrakeLightIndic)
%#codegen
TargetBrake_b = false;
TargetVxG = single(0);
TargetVyG = single(0);

if (ID>0)&&(ID<100)
    if BrakeLightIndic(ID)==2
        TargetBrake_b = true;
    end
    TargetVxG = VxG(ID);
    TargetVyG = VyG(ID);
end
